simulink model "model"  (R2024a)
settings: Solver=ode4  StartTime=0.0  StopTime=6000  FixedStep=0.1  MaxStep=1  RelTol=1e-6  AbsTol=1e-9
undefined symbols (not defined in the file or in its folder): constants, P0, q0, rECI0, rSCI0, sensors, vECI0, vSCI0, w0
libraries: vrlib x2, aerolibatmos2 x1
settings Model: Creator=harryzhao  LastModifiedBy=harryzhao

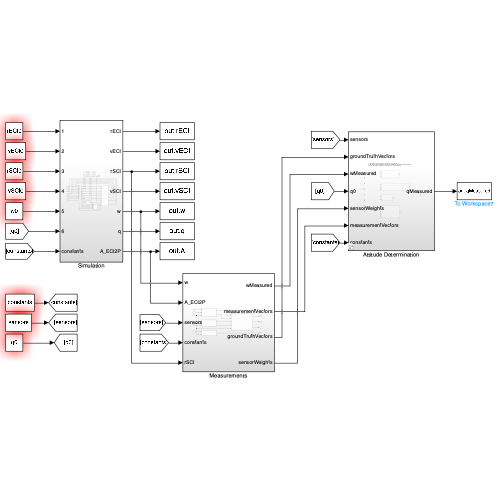
[thumbnail: Simulink's stored preview of the top-level diagram]
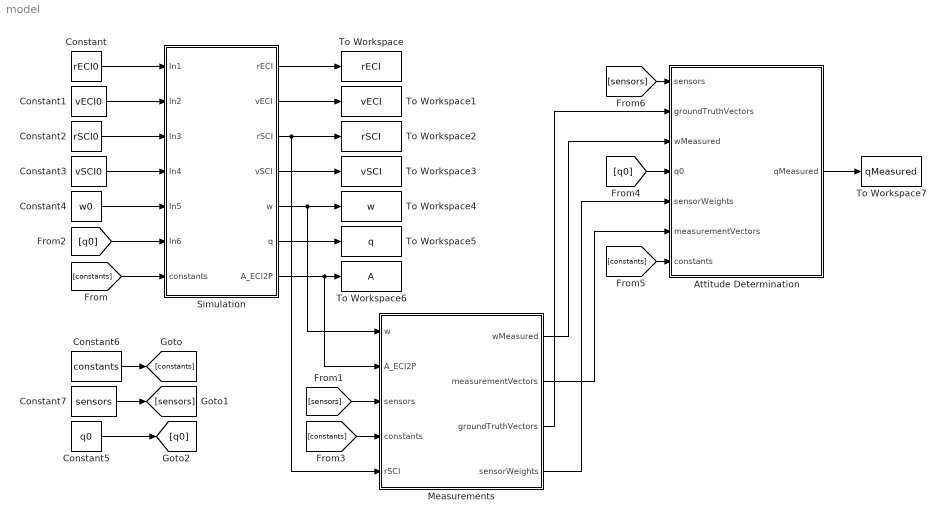
== system model ==
  Attitude Determination : Subsystem  Variant=on
  Constant : Constant  Value=rECI0
  Constant1 : Constant  Value=vECI0
  Constant2 : Constant  Value=rSCI0
  Constant3 : Constant  Value=vSCI0
  Constant4 : Constant  Value=w0
  Constant5 : Constant  Value=q0
  Constant6 : Constant  Value=constants  OutDataTypeStr=Bus: constants_bus
  Constant7 : Constant  Value=sensors  OutDataTypeStr=Bus: sensors_bus
  Measurements : Subsystem
  Simulation : Subsystem
  To Workspace : ToWorkspace  VariableName=rECI  SaveFormat=Timeseries  SampleTime=-1
  To Workspace1 : ToWorkspace  VariableName=vECI  SaveFormat=Timeseries  SampleTime=-1
  To Workspace2 : ToWorkspace  VariableName=rSCI  SaveFormat=Timeseries  SampleTime=-1
  To Workspace3 : ToWorkspace  VariableName=vSCI  SaveFormat=Timeseries  SampleTime=-1
  To Workspace4 : ToWorkspace  VariableName=w  SaveFormat=Timeseries  SampleTime=-1
  To Workspace5 : ToWorkspace  VariableName=q  SaveFormat=Timeseries  SampleTime=-1
  To Workspace6 : ToWorkspace  VariableName=A  SaveFormat=Timeseries  SampleTime=-1
  To Workspace7 : ToWorkspace  VariableName=qMeasured  SaveFormat=Timeseries  SampleTime=-1
  wires:
  Constant2/1 -> Simulation/3(In3)
  Measurements/4(sensorWeights) -> Attitude Determination/5(sensorWeights)
  Constant4/1 -> Simulation/5(In5)
  Measurements/2(measurementVectors) -> Attitude Determination/6(measurementVectors)
  Constant3/1 -> Simulation/4(In4)
  Simulation/1(rECI) -> To Workspace/1
  Simulation/2(vECI) -> To Workspace1/1
  Simulation/3(rSCI) -> Measurements/5(rSCI), To Workspace2/1
  Simulation/4(vSCI) -> To Workspace3/1
  Simulation/5(w) -> Measurements/1(w), To Workspace4/1
  Simulation/6(q) -> To Workspace5/1
  Simulation/7(A_ECI2P) -> Measurements/2(A_ECI2P), To Workspace6/1
  Measurements/1(wMeasured) -> Attitude Determination/3(wMeasured)
  Measurements/3(groundTruthVectors) -> Attitude Determination/2(groundTruthVectors)
  Attitude Determination/1(qMeasured) -> To Workspace7/1
  Constant/1 -> Simulation/1(In1)
  Constant1/1 -> Simulation/2(In2)
  [q0] -> Simulation/6(In6)
  [constants] -> Simulation/7(constants)
  Constant6/1 -> [constants]
  Constant7/1 -> [sensors]
  Constant5/1 -> [q0]
  [sensors] -> Measurements/3(sensors)
  [constants] -> Measurements/4(constants)
  [q0] -> Attitude Determination/4(q0)
  [constants] -> Attitude Determination/7(constants)
  [sensors] -> Attitude Determination/1(sensors)

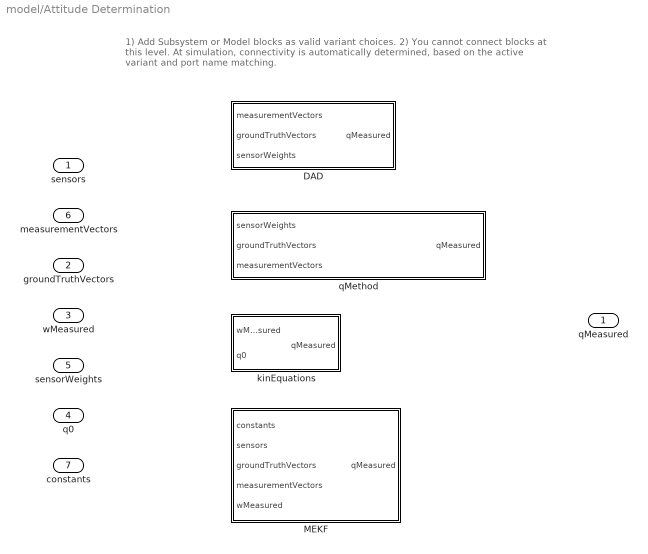
== system model/Attitude Determination ==
  note: 1) Add Subsystem or Model blocks as valid variant choices.
      | 2) You cannot connect blocks at this level. At simulation, connectivity is automatically
      | determined, based on the active variant and port name matching.
  sensors : Inport
  groundTruthVectors : Inport  Port=2
  wMeasured : Inport  Port=3
  q0 : Inport  Port=4
  sensorWeights : Inport  Port=5
  measurementVectors : Inport  Port=6
  constants : Inport  Port=7
  DAD : Subsystem  VariantControl="measType==\"dad\""
  MEKF : Subsystem  VariantControl="measType==\"MEKF\""
  kinEquations : Subsystem  VariantControl="measType==\"kin\""
  qMethod : Subsystem  VariantControl="measType==\"q\""
  qMeasured : Outport

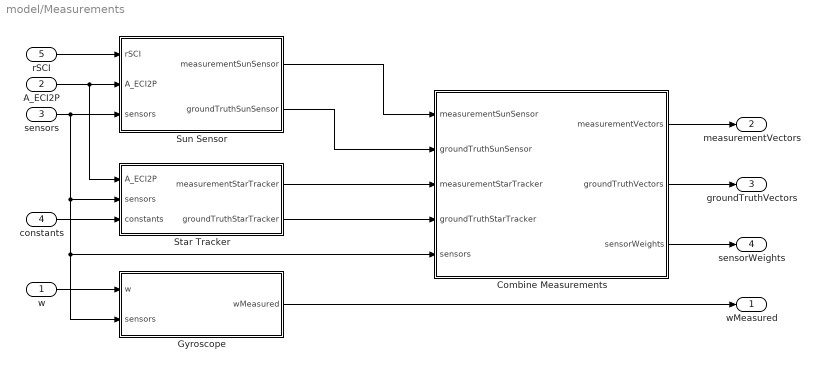
== system model/Measurements ==
  w : Inport
  A_ECI2P : Inport  Port=2
  sensors : Inport  Port=3
  constants : Inport  Port=4
  rSCI : Inport  Port=5
  Combine Measurements : MATLAB Function  TreatAsAtomicUnit=on
  Gyroscope : MATLAB Function  TreatAsAtomicUnit=on
  Star Tracker : MATLAB Function  TreatAsAtomicUnit=on
  Sun Sensor : MATLAB Function  TreatAsAtomicUnit=on
  wMeasured : Outport
  measurementVectors : Outport  Port=2
  groundTruthVectors : Outport  Port=3
  sensorWeights : Outport  Port=4
  wires:
  rSCI/1 -> Sun Sensor/1(rSCI)
  A_ECI2P/1 -> Star Tracker/1(A_ECI2P), Sun Sensor/2(A_ECI2P)
  sensors/1 -> Gyroscope/2(sensors), Combine Measurements/5(sensors), Star Tracker/2(sensors), Sun Sensor/3(sensors)
  constants/1 -> Star Tracker/3(constants)
  w/1 -> Gyroscope/1(w)
  Gyroscope/1(wMeasured) -> wMeasured/1
  Sun Sensor/2(groundTruthSunSensor) -> Combine Measurements/2(groundTruthSunSensor)
  Sun Sensor/1(measurementSunSensor) -> Combine Measurements/1(measurementSunSensor)
  Star Tracker/1(measurementStarTracker) -> Combine Measurements/3(measurementStarTracker)
  Star Tracker/2(groundTruthStarTracker) -> Combine Measurements/4(groundTruthStarTracker)
  Combine Measurements/1(measurementVectors) -> measurementVectors/1
  Combine Measurements/2(groundTruthVectors) -> groundTruthVectors/1
  Combine Measurements/3(sensorWeights) -> sensorWeights/1

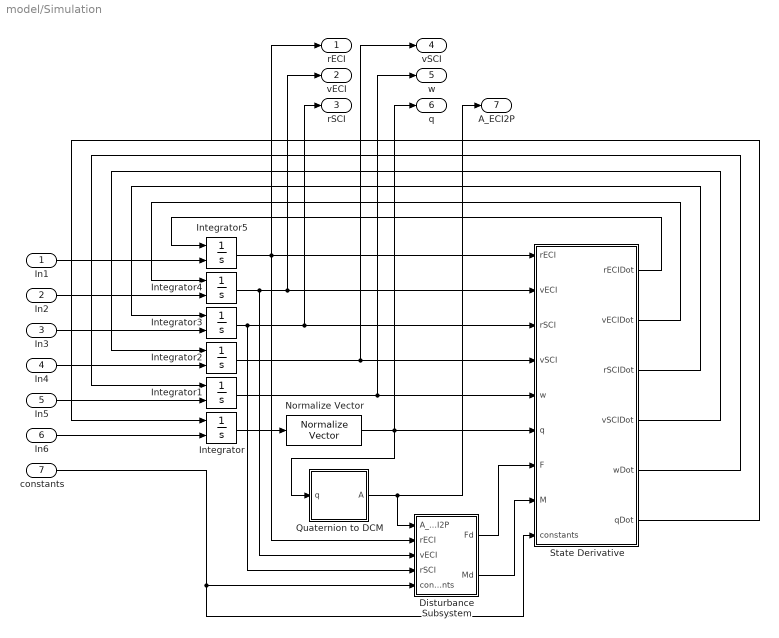
== system model/Simulation ==
  In1 : Inport
  In2 : Inport  Port=2
  In3 : Inport  Port=3
  In4 : Inport  Port=4
  In5 : Inport  Port=5
  In6 : Inport  Port=6
  constants : Inport  Port=7
  Disturbance Subsystem : Subsystem
  Integrator{,1..5} (6 alike) : Integrator  InitialConditionSource=external
  Normalize Vector : vrlib/Utilities/Normalize Vector  maxzero=0
  Quaternion to DCM : MATLAB Function  TreatAsAtomicUnit=on
  State Derivative : MATLAB Function  TreatAsAtomicUnit=on
  rECI : Outport
  vECI : Outport  Port=2
  rSCI : Outport  Port=3
  vSCI : Outport  Port=4
  w : Outport  Port=5
  q : Outport  Port=6
  A_ECI2P : Outport  Port=7
  wires:
  Disturbance Subsystem/1(Fd) -> State Derivative/7(F)
  Integrator3/1 -> rSCI/1, State Derivative/3(rSCI), Disturbance Subsystem/4(rSCI)
  Integrator2/1 -> vSCI/1, State Derivative/4(vSCI)
  Integrator/1 -> Normalize Vector/1
  In2/1 -> Integrator4/2
  Integrator5/1 -> rECI/1, State Derivative/1(rECI), Disturbance Subsystem/2(rECI)
  Normalize Vector/1 -> Quaternion to DCM/1(q), q/1, State Derivative/6(q)
  constants/1 -> Disturbance Subsystem/5(constants), State Derivative/9(constants)
  Integrator4/1 -> vECI/1, State Derivative/2(vECI), Disturbance Subsystem/3(vECI)
  In3/1 -> Integrator3/2
  State Derivative/3(rSCIDot) -> Integrator3/1
  State Derivative/1(rECIDot) -> Integrator5/1
  Quaternion to DCM/1(A) -> A_ECI2P/1, Disturbance Subsystem/1(A_ECI2P)
  State Derivative/4(vSCIDot) -> Integrator2/1
  Disturbance Subsystem/2(Md) -> State Derivative/8(M)
  State Derivative/6(qDot) -> Integrator/1
  Integrator1/1 -> w/1, State Derivative/5(w)
  State Derivative/5(wDot) -> Integrator1/1
  In4/1 -> Integrator2/2
  State Derivative/2(vECIDot) -> Integrator4/1
  In6/1 -> Integrator/2
  In5/1 -> Integrator1/2
  In1/1 -> Integrator5/2

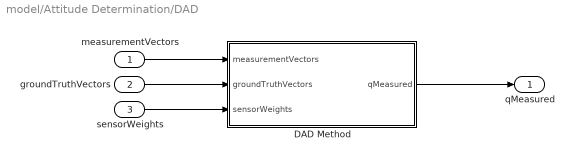
== system model/Attitude Determination/DAD ==
  measurementVectors : Inport
  groundTruthVectors : Inport  Port=2
  sensorWeights : Inport  Port=3
  DAD Method : Subsystem  Variant=on
  qMeasured : Outport
  wires:
  groundTruthVectors/1 -> DAD Method/2(groundTruthVectors)
  measurementVectors/1 -> DAD Method/1(measurementVectors)
  DAD Method/1(qMeasured) -> qMeasured/1
  sensorWeights/1 -> DAD Method/3(sensorWeights)

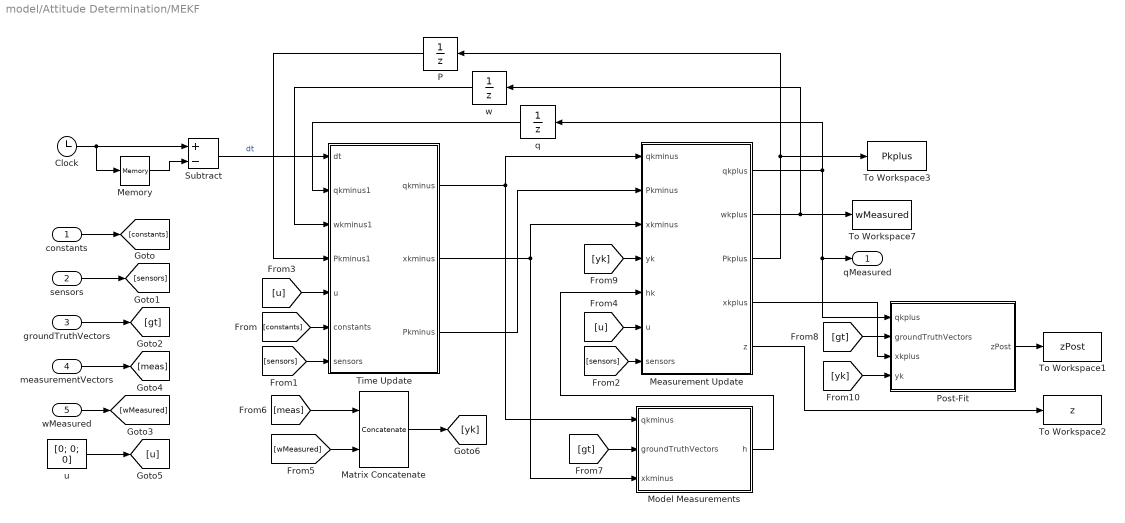
== system model/Attitude Determination/MEKF ==
  constants : Inport
  sensors : Inport  Port=2
  groundTruthVectors : Inport  Port=3
  measurementVectors : Inport  Port=4
  wMeasured : Inport  Port=5
  Clock : Clock
  Matrix Concatenate : Concatenate  Mode=Multidimensional array  ConcatenateDimension=2
  Measurement Update : MATLAB Function  TreatAsAtomicUnit=on
  Memory : Memory
  Model Measurements : Subsystem
  P : UnitDelay  InitialCondition=P0  SampleTime=-1  HasFrameUpgradeWarning=on
  Post-Fit : Subsystem
  Subtract : Sum  Inputs=+-
  Time Update : MATLAB Function  TreatAsAtomicUnit=on
  To Workspace1 : ToWorkspace  VariableName=zPost  SaveFormat=Timeseries  SampleTime=-1
  To Workspace2 : ToWorkspace  VariableName=z  SaveFormat=Timeseries  SampleTime=-1
  To Workspace3 : ToWorkspace  VariableName=Pkplus  SaveFormat=Timeseries  SampleTime=-1
  To Workspace7 : ToWorkspace  VariableName=wMeasured  SaveFormat=Timeseries  SampleTime=-1
  q : UnitDelay  InitialCondition=q0  SampleTime=-1  HasFrameUpgradeWarning=on
  u : Constant  Value=[0; 0; 0]
  w : UnitDelay  InitialCondition=w0'  SampleTime=-1  HasFrameUpgradeWarning=on
  qMeasured : Outport
  wires:
  Clock/1 -> Memory/1, Subtract/1
  Memory/1 -> Subtract/2
  Time Update/2(xkminus) -> Measurement Update/3(xkminus), Model Measurements/3(xkminus)
  Subtract/1 -> Time Update/1(dt)  "dt"
  Time Update/1(qkminus) -> Measurement Update/1(qkminus), Model Measurements/1(qkminus)
  Time Update/3(Pkminus) -> Measurement Update/2(Pkminus)
  Model Measurements/1(h) -> Measurement Update/5(hk)
  Measurement Update/1(qkplus) -> Post-Fit/1(qkplus), qMeasured/1, q/1
  Measurement Update/2(wkplus) -> To Workspace7/1, w/1
  Measurement Update/3(Pkplus) -> P/1, To Workspace3/1
  P/1 -> Time Update/4(Pkminus1)
  w/1 -> Time Update/3(wkminus1)
  q/1 -> Time Update/2(qkminus1)
  Measurement Update/4(xkplus) -> Post-Fit/3(xkplus)
  constants/1 -> [constants]
  sensors/1 -> [sensors]
  [constants] -> Time Update/6(constants)
  [sensors] -> Time Update/7(sensors)
  [sensors] -> Measurement Update/7(sensors)
  u/1 -> [u]
  [u] -> Time Update/5(u)
  [u] -> Measurement Update/6(u)
  wMeasured/1 -> [wMeasured]
  [wMeasured] -> Matrix Concatenate/2
  measurementVectors/1 -> [meas]
  [meas] -> Matrix Concatenate/1
  groundTruthVectors/1 -> [gt]
  [gt] -> Model Measurements/2(groundTruthVectors)
  [gt] -> Post-Fit/2(groundTruthVectors)
  Measurement Update/5(z) -> To Workspace2/1
  Matrix Concatenate/1 -> [yk]
  [yk] -> Measurement Update/4(yk)
  [yk] -> Post-Fit/4(yk)
  Post-Fit/1(zPost) -> To Workspace1/1

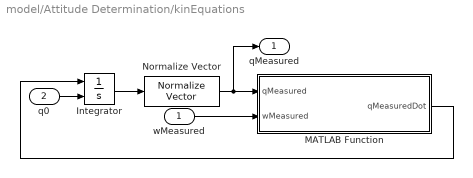
== system model/Attitude Determination/kinEquations ==
  wMeasured : Inport
  q0 : Inport  Port=2
  Integrator : Integrator  InitialConditionSource=external
  MATLAB Function : MATLAB Function  TreatAsAtomicUnit=on
  Normalize Vector : vrlib/Utilities/Normalize Vector  maxzero=0
  qMeasured : Outport
  wires:
  wMeasured/1 -> MATLAB Function/2(wMeasured)
  MATLAB Function/1(qMeasuredDot) -> Integrator/1
  q0/1 -> Integrator/2
  Normalize Vector/1 -> qMeasured/1, MATLAB Function/1(qMeasured)
  Integrator/1 -> Normalize Vector/1

== system model/Attitude Determination/qMethod ==
  sensorWeights : Inport
  groundTruthVectors : Inport  Port=2
  measurementVectors : Inport  Port=3
  MATLAB Function : MATLAB Function  TreatAsAtomicUnit=on
  qMeasured : Outport
  wires:
  MATLAB Function/1(qMeasured) -> qMeasured/1
  sensorWeights/1 -> MATLAB Function/3(sensorWeights)
  groundTruthVectors/1 -> MATLAB Function/2(groundTruthVectors)
  measurementVectors/1 -> MATLAB Function/1(measurementVectors)

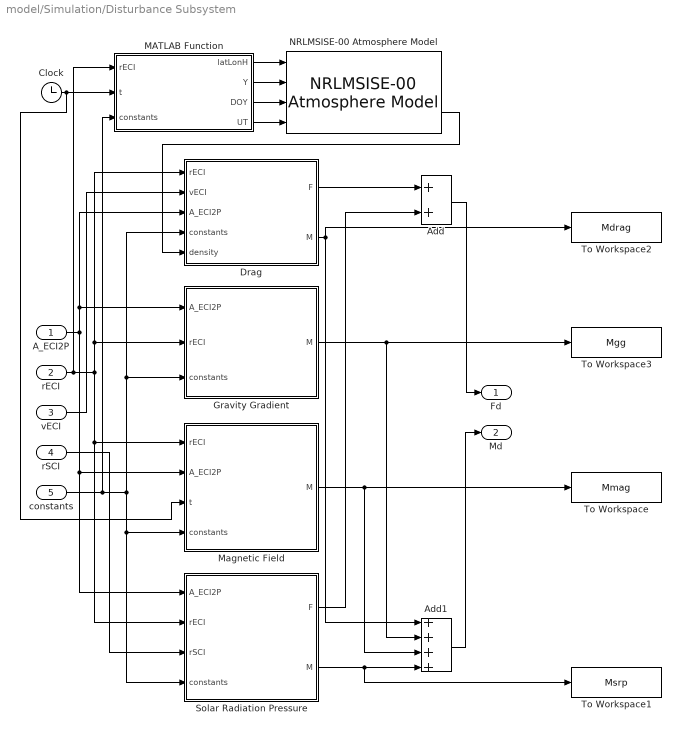
== system model/Simulation/Disturbance Subsystem ==
  A_ECI2P : Inport
  rECI : Inport  Port=2
  vECI : Inport  Port=3
  rSCI : Inport  Port=4
  constants : Inport  Port=5
  Add : Sum
  Add1 : Sum  Inputs=++++
  Clock : Clock
  Drag : MATLAB Function  TreatAsAtomicUnit=on
  Gravity Gradient : MATLAB Function  TreatAsAtomicUnit=on
  MATLAB Function : MATLAB Function  TreatAsAtomicUnit=on
  Magnetic Field : MATLAB Function  TreatAsAtomicUnit=on
  NRLMSISE-00 Atmosphere Model : aerolibatmos2/NRLMSISE-00 Atmosphere Model  units=Metric (MKS)  lst_input=off  flux_ap_input=off  flags_input=Internal  flags=ones(1,23)  oxygen_in=off  action=Warning
  Solar Radiation Pressure : MATLAB Function  TreatAsAtomicUnit=on
  To Workspace : ToWorkspace  VariableName=Mmag  SaveFormat=Timeseries  SampleTime=-1
  To Workspace1 : ToWorkspace  VariableName=Msrp  SaveFormat=Timeseries  SampleTime=-1
  To Workspace2 : ToWorkspace  VariableName=Mdrag  SaveFormat=Timeseries  SampleTime=-1
  To Workspace3 : ToWorkspace  VariableName=Mgg  SaveFormat=Timeseries  SampleTime=-1
  Fd : Outport
  Md : Outport  Port=2
  wires:
  Gravity Gradient/1(M) -> To Workspace3/1, Add1/2
  Drag/2(M) -> To Workspace2/1, Add1/1
  Solar Radiation Pressure/1(F) -> Add/2
  Drag/1(F) -> Add/1
  Add/1 -> Fd/1
  Add1/1 -> Md/1
  A_ECI2P/1 -> Magnetic Field/2(A_ECI2P), Solar Radiation Pressure/1(A_ECI2P), Drag/3(A_ECI2P), Gravity Gradient/1(A_ECI2P)
  rECI/1 -> MATLAB Function/1(rECI), Solar Radiation Pressure/2(rECI), Magnetic Field/1(rECI), Gravity Gradient/2(rECI), Drag/1(rECI)
  vECI/1 -> Drag/2(vECI)
  rSCI/1 -> Solar Radiation Pressure/3(rSCI)
  Solar Radiation Pressure/2(M) -> To Workspace1/1, Add1/4
  Magnetic Field/1(M) -> To Workspace/1, Add1/3
  constants/1 -> MATLAB Function/3(constants), Magnetic Field/4(constants), Solar Radiation Pressure/4(constants), Gravity Gradient/3(constants), Drag/4(constants)
  MATLAB Function/2(Y) -> NRLMSISE-00 Atmosphere Model/2
  MATLAB Function/3(DOY) -> NRLMSISE-00 Atmosphere Model/3
  MATLAB Function/4(UT) -> NRLMSISE-00 Atmosphere Model/4
  MATLAB Function/1(latLonH) -> NRLMSISE-00 Atmosphere Model/1
  NRLMSISE-00 Atmosphere Model/2 -> Drag/5(density)
  Clock/1 -> MATLAB Function/2(t), Magnetic Field/3(t)

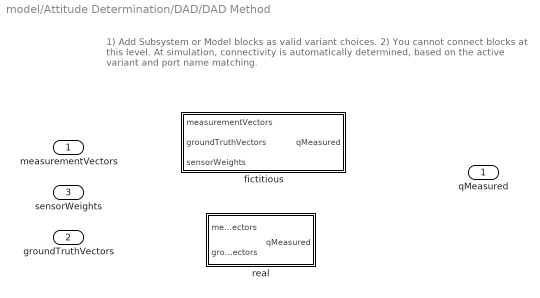
== system model/Attitude Determination/DAD/DAD Method ==
  note: 1) Add Subsystem or Model blocks as valid variant choices.
      | 2) You cannot connect blocks at this level. At simulation, connectivity is automatically
      | determined, based on the active variant and port name matching.
  measurementVectors : Inport
  groundTruthVectors : Inport  Port=2
  sensorWeights : Inport  Port=3
  fictitious : Subsystem  VariantControl=useFict == true
  real : Subsystem  VariantControl=useFict == false
  qMeasured : Outport

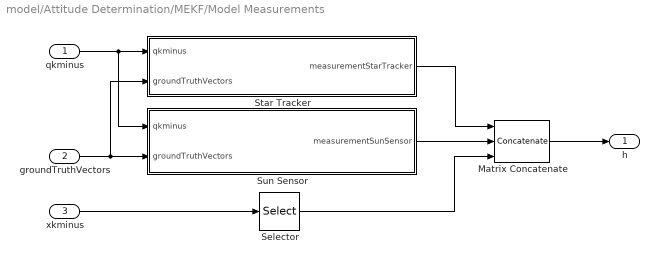
== system model/Attitude Determination/MEKF/Model Measurements ==
  qkminus : Inport
  groundTruthVectors : Inport  Port=2
  xkminus : Inport  Port=3
  Matrix Concatenate : Concatenate  NumInputs=3  Mode=Multidimensional array  ConcatenateDimension=2
  Selector : Selector  NumberOfDimensions=2  InputPortWidth=3  IndexOptions=Index vector (dialog),Index vector (dialog)  Indices=[4:6],1  OutputSizes=1,1
  Star Tracker : MATLAB Function  TreatAsAtomicUnit=on
  Sun Sensor : MATLAB Function  TreatAsAtomicUnit=on
  h : Outport
  wires:
  groundTruthVectors/1 -> Star Tracker/2(groundTruthVectors), Sun Sensor/2(groundTruthVectors)
  qkminus/1 -> Sun Sensor/1(qkminus), Star Tracker/1(qkminus)
  Star Tracker/1(measurementStarTracker) -> Matrix Concatenate/1
  Sun Sensor/1(measurementSunSensor) -> Matrix Concatenate/2
  Matrix Concatenate/1 -> h/1
  xkminus/1 -> Selector/1
  Selector/1 -> Matrix Concatenate/3

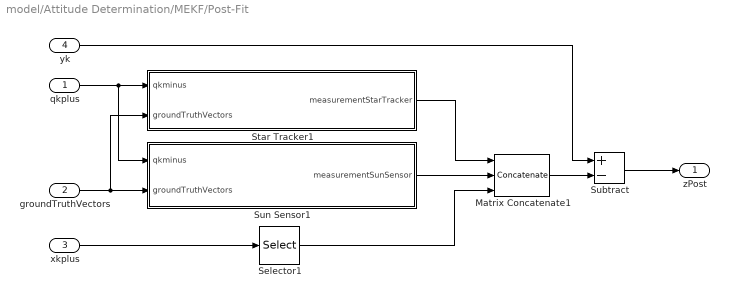
== system model/Attitude Determination/MEKF/Post-Fit ==
  qkplus : Inport
  groundTruthVectors : Inport  Port=2
  xkplus : Inport  Port=3
  yk : Inport  Port=4
  Matrix Concatenate1 : Concatenate  NumInputs=3  Mode=Multidimensional array  ConcatenateDimension=2
  Selector1 : Selector  NumberOfDimensions=2  InputPortWidth=3  IndexOptions=Index vector (dialog),Index vector (dialog)  Indices=[4:6],1  OutputSizes=1,1
  Star Tracker1 : MATLAB Function  TreatAsAtomicUnit=on
  Subtract : Sum  Inputs=+-
  Sun Sensor1 : MATLAB Function  TreatAsAtomicUnit=on
  zPost : Outport
  wires:
  Subtract/1 -> zPost/1
  qkplus/1 -> Sun Sensor1/1(qkminus), Star Tracker1/1(qkminus)
  Selector1/1 -> Matrix Concatenate1/3
  xkplus/1 -> Selector1/1
  groundTruthVectors/1 -> Star Tracker1/2(groundTruthVectors), Sun Sensor1/2(groundTruthVectors)
  Star Tracker1/1(measurementStarTracker) -> Matrix Concatenate1/1
  Sun Sensor1/1(measurementSunSensor) -> Matrix Concatenate1/2
  Matrix Concatenate1/1 -> Subtract/2
  yk/1 -> Subtract/1

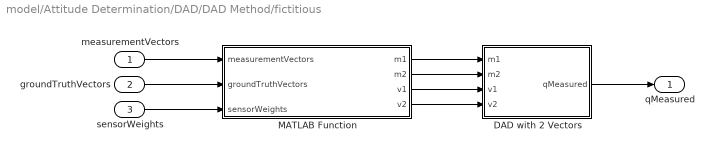
== system model/Attitude Determination/DAD/DAD Method/fictitious ==
  measurementVectors : Inport
  groundTruthVectors : Inport  Port=2
  sensorWeights : Inport  Port=3
  DAD with 2 Vectors : MATLAB Function  TreatAsAtomicUnit=on
  MATLAB Function : MATLAB Function  TreatAsAtomicUnit=on
  qMeasured : Outport
  wires:
  measurementVectors/1 -> MATLAB Function/1(measurementVectors)
  groundTruthVectors/1 -> MATLAB Function/2(groundTruthVectors)
  MATLAB Function/1(m1) -> DAD with 2 Vectors/1(m1)
  MATLAB Function/2(m2) -> DAD with 2 Vectors/2(m2)
  MATLAB Function/3(v1) -> DAD with 2 Vectors/3(v1)
  MATLAB Function/4(v2) -> DAD with 2 Vectors/4(v2)
  DAD with 2 Vectors/1(qMeasured) -> qMeasured/1
  sensorWeights/1 -> MATLAB Function/3(sensorWeights)

== system model/Attitude Determination/DAD/DAD Method/real ==
  measurementVectors : Inport
  groundTruthVectors : Inport  Port=2
  MATLAB Function : MATLAB Function  TreatAsAtomicUnit=on
  qMeasured : Outport
  wires:
  measurementVectors/1 -> MATLAB Function/1(measurementVectors)
  groundTruthVectors/1 -> MATLAB Function/2(groundTruthVectors)
  MATLAB Function/1(qMeasured) -> qMeasured/1

== matlab function model/Attitude Determination/DAD/DAD Method/fictitious/DAD with 2 Vectors ==
  data: m1 input; qMeasured output; m2 input; v1 input; v2 input
function qMeasured = DAD2Vec(m1, m2, v1, v2)
% Implement the Deterministic Atittude Determination algorithm
% Inputs:
% - m1, m2: measured vectors
% - v1, v2: ground truth vector
% Outputs:
% - A: DCM between principal axes and ECI

pm = m1;
cross_qm = cross(m1, m2);
qm = cross_qm/norm(cross_qm);
rm = cross(pm, qm);

pv = v1;
cross_qv = cross(v1, v2);
qv = cross_qv/norm(cross_qv);
rv = cross(pv,qv);

M = [pm qm rm];
V = [pv qv rv];
A = M / V;
qMeasured = A2q(A);
end

== matlab function model/Attitude Determination/qMethod/MATLAB Function ==
  data: measurementVectors input; groundTruthVectors input; sensorWeights input; qMeasured output size=[4, 1]
function qMeasured = qMethod(measurementVectors, groundTruthVectors, sensorWeights)
    % Implement the Deterministic q method
    % Inputs:
    % - m: measured vectors
    % - v: ground truth vector
    % - w: weights of sensor measurements
    % Outputs:
    % - A: DCM between principal axes and ECI

    % Get data from sensors
    m = measurementVectors;
    v = groundTruthVectors;
    w = sensorWeights;
    % m = ones(3); v = ones(3); w = ones(3);


    U = sqrt(w) .* v;
    W = sqrt(w) .* m;

    B = W * U';
    S = B + B';
    Z = [B(2,3)-B(3,2), B(3,1)-B(1,3), B(1,2)-B(2,1)]';
    sigma = trace(B);

    K = [S - eye(size(S))*sigma, Z;
            Z', sigma];

    [V, lamda] = eig(K);

    [~, nMax] = max(diag(lamda));

    qMeasured = V(:, nMax);
    qMeasured = A2q(q2A(qMeasured));
end

== matlab function model/Attitude Determination/kinEquations/MATLAB Function ==
  data: qMeasured input; qMeasuredDot output; wMeasured input
function qMeasuredDot = kinQuats(qMeasured, wMeasured)
    
    w = wMeasured;

    sigma = [0, w(3), -w(2), w(1); ...
        -w(3), 0, w(1), w(2); ...
        w(2), -w(1), 0, w(3); ...
        -w(1), -w(2), -w(3), 0];
    qMeasuredDot = 0.5 * sigma * qMeasured;
end

== matlab function model/Attitude Determination/DAD/DAD Method/fictitious/MATLAB Function ==
  data: measurementVectors input; m1 output; groundTruthVectors input; m2 output; v1 output; v2 output; sensorWeights input
function [m1, m2, v1, v2] = getMeasurementsFict(measurementVectors, groundTruthVectors, sensorWeights)
    [~, indBest2Sensors] = maxk(sensorWeights, 2);
    mVec = measurementVectors(:,indBest2Sensors);
    vVec = groundTruthVectors(:,indBest2Sensors);

    m1 = (mVec(:,1) + mVec(:,2))/2;
    m2 = (mVec(:,1) - mVec(:,2))/2;
    v1 = (vVec(:,1) + vVec(:,2))/2;
    v2 = ((vVec(:,1) - vVec(:,2))/2);

    m1 = m1 / norm(m1);
    m2 = m2 / norm(m2);
    v1 = v1 / norm(v1);
    v2 = v2 / norm(v2);
end

== matlab function model/Attitude Determination/DAD/DAD Method/real/MATLAB Function ==
  data: measurementVectors input; qMeasured output; groundTruthVectors input
function qMeasured = DAD(measurementVectors, groundTruthVectors)
    % Implement the Deterministic Atittude Determination algorithm
    % Inputs:
    % - m: measured vectors ([m1 m2 . . . ])
    % - v: ground truth vector ([v1 v2 . . . ])
    % Outputs:
    % - A: DCM between principal axes and ECI

    A = measurementVectors * pinv(groundTruthVectors);
    qMeasured = A2q(A);
end

== matlab function model/Measurements/Sun Sensor ==
  settings: updateMethod=DISCRETE
  data: rSCI input; A_ECI2P input; sensors input; measurementSunSensor output; groundTruthSunSensor output
function [measurementSunSensor,groundTruthSunSensor] = sunSensor(rSCI, A_ECI2P, sensors)
    % Get sensor measurement without noise
    rSunSensors = A_ECI2P * rSCI;
    rSunSensors = normVec(rSunSensors);
    
    % Add noise
    % measurementSunSensor = addVectorNoise(rSunSensors, sensors.sunError);
    measurementSunSensor = addNoise(rSunSensors, sensors.sunError);
    measurementSunSensor = normVec(measurementSunSensor);

    % Get groud truth
    groundTruthSunSensor = normVec(rSCI);

end

== matlab function model/Measurements/Star Tracker ==
  settings: updateMethod=DISCRETE
  data: A_ECI2P input; sensors input; constants input; measurementStarTracker output; groundTruthStarTracker output
function [measurementStarTracker, groundTruthStarTracker] = starTracker(A_ECI2P, sensors, constants)
    % Get sensor measurement without noise (body axes)
    % numStars = sensors.numStars;
    numStars = 10;
    rStarBody = zeros([3, numStars*2]);
    for i = 1:numStars
        theta = deg2rad(randi([0 359], 1));
        phi = 2*sensors.trackerFOV *rand(1) - sensors.trackerFOV;
        rStarBody(:,i) = [cos(theta)*sin(phi); cos(phi); sin(theta)*sin(phi)];
        rStarBody(:,i+numStars) = [cos(theta)*sin(phi); -cos(phi); sin(theta)*sin(phi)];
    end

    % Convert to principal axes
    rStarP = constants.A_Body2P * rStarBody;

    measurementStarTracker = addNoise(rStarP, sensors.trackerError);
    measurementStarTracker = normVec(measurementStarTracker);

    % Get ground truth data
    groundTruthStarTracker = A_ECI2P' * rStarP;
end

== matlab function model/Measurements/Gyroscope ==
  settings: updateMethod=DISCRETE
  data: w input; sensors input; wMeasured output
function wMeasured = gyro(w, sensors)
    % Add noise to gyro measurements
    wMeasured = addNoise(w, sensors.gyroError, sensors.gyroBias);
end

== matlab function model/Measurements/Combine Measurements ==
  data: measurementSunSensor input; groundTruthSunSensor input; measurementStarTracker input; groundTruthStarTracker input; sensors input; measurementVectors output; groundTruthVectors output; sensorWeights output
function [measurementVectors, groundTruthVectors, sensorWeights] = concatenateMeasurements(measurementSunSensor, groundTruthSunSensor, measurementStarTracker, groundTruthStarTracker, sensors)
    % Initialize
    vectorSize = size(measurementStarTracker, 2) + size(measurementSunSensor, 2);

    % Concatenate such that we have [starTracker, sunSensor]
    measurementVectors = [measurementStarTracker, measurementSunSensor];
    groundTruthVectors = [groundTruthStarTracker, groundTruthSunSensor];
    
    % Get sensor weighting
    sensorWeights = [ones([1, vectorSize-1])*sensors.weights(1), sensors.weights(2)];
end

== matlab function model/Attitude Determination/MEKF/Post-Fit/Star Tracker1 ==
  settings: updateMethod=DISCRETE
  data: qkminus input; groundTruthVectors input; measurementStarTracker output
function measurementStarTracker = starTracker(qkminus,groundTruthVectors)
    % Extract information
    A_ECI2P = q2A(qkminus);
    rStarECI = groundTruthVectors(:,1:end-1);
    rStarP = A_ECI2P * rStarECI;

    measurementStarTracker = normVec(rStarP);
end

== matlab function model/Attitude Determination/MEKF/Post-Fit/Sun Sensor1 ==
  settings: updateMethod=DISCRETE
  data: qkminus input; groundTruthVectors input; measurementSunSensor output
function measurementSunSensor = sunSensor(qkminus,groundTruthVectors)
    % Get modeled parameters
    rSCI = groundTruthVectors(:,end);
    A_ECI2P = q2A(qkminus);

    % Get sensor measurement without noise
    rSunSensors = A_ECI2P * rSCI;
    measurementSunSensor = normVec(rSunSensors);
end

== matlab function model/Attitude Determination/MEKF/Measurement Update ==
  data: qkminus input; Pkminus input; xkminus input; yk input; hk input; u input; sensors input; qkplus output; wkplus output; Pkplus output; xkplus output; z output
function [qkplus,wkplus,Pkplus,xkplus,z] = measurementUpdate(qkminus, Pkminus, xkminus, yk, hk, u, sensors)
    % Get R
    numVectMeasurements = size(hk,2)-1;
    R = diag([repelem(sensors.trackerError, 3*(numVectMeasurements-1)), repelem(sensors.sunError, 3), repelem(sensors.gyroError, 3)]).^2;

    % Compute residual
    z = yk - hk;

    % Adjust yk and hk vectors
    yk = yk(:);
    hk = hk(:);
    
    % Get Hk
    Hk = zeros([3*(numVectMeasurements+1), 6]);
    for n = 1:3:(3*numVectMeasurements)
        Hk_vect = crossMatrix(hk(n:n+2));
        Hk(n:n+2,:) = [Hk_vect, zeros(3)];
    end
    Hk(end-2:end,:) = [zeros(3), eye(3)];
    Kk = (Pkminus * Hk') / (Hk * Pkminus * Hk' + R);
    xkplus = xkminus + Kk * (yk - hk);
    Pkplus = Pkminus - Kk * Hk * Pkminus;
    wkplus = xkplus(4:6);
    ax = xkplus(1); ay = xkplus(2); az = xkplus(3);

    % Attitude update
    qkplus = [1, az/2, -ay/2, ax/2; ...
        -az/2, 1, ax/2, ay/2; ...
        ay/2, -ax/2, 1, az/2; ...
        -ax/2, -ay/2, -az/2, 1] * qkminus;
end

== matlab function model/Simulation/Quaternion to DCM ==
  data: q input size=[4 1]; A output
function A = q2A(q)
    q1 = q(1); q2 = q(2); q3 = q(3); q0 = q(4);
    A = [(q0^2 + q1^2 - q2^2 - q3^2) (2 * q1 * q2 + 2 * q0 * q3) (2 * q1 * q3 - 2 * q0 * q2); ...
        (2 * q1 * q2 - 2 * q0 * q3) (q0^2 - q1^2 + q2^2 - q3^2) (2 * q2 * q3 + 2 * q0 * q1); ...
        (2 * q1 * q3 + 2 * q0 * q2) (2 * q2 * q3 - 2 * q0 * q1) (q0^2 - q1^2 - q2^2 + q3^2)];
end

== matlab function model/Attitude Determination/MEKF/Model Measurements/Star Tracker ==
  settings: updateMethod=DISCRETE
  data: qkminus input; groundTruthVectors input; measurementStarTracker output
function measurementStarTracker = starTracker(qkminus,groundTruthVectors)
    % Extract information
    A_ECI2P = q2A(qkminus);
    rStarECI = groundTruthVectors(:,1:end-1);
    rStarP = A_ECI2P * rStarECI;

    measurementStarTracker = normVec(rStarP);
end

== matlab function model/Attitude Determination/MEKF/Model Measurements/Sun Sensor ==
  settings: updateMethod=DISCRETE
  data: qkminus input; groundTruthVectors input; measurementSunSensor output
function measurementSunSensor = sunSensor(qkminus,groundTruthVectors)
    % Get modeled parameters
    rSCI = groundTruthVectors(:,end);
    A_ECI2P = q2A(qkminus);

    % Get sensor measurement without noise
    rSunSensors = A_ECI2P * rSCI;
    measurementSunSensor = normVec(rSunSensors);
end

== matlab function model/Attitude Determination/MEKF/Time Update ==
  data: dt input; qkminus output size=[4, 1]; qkminus1 input; wkminus1 input; Pkminus1 input; u input; constants input; sensors input; xkminus output size=[6, 1]; Pkminus output size=[6, 6]
function [qkminus, xkminus, Pkminus] = timeUpdate(dt, qkminus1, wkminus1, Pkminus1, u, constants, sensors)
    % MEKF, only time update implemented

    % Get values
    Ix = constants.Ix; Iy = constants.Iy; Iz = constants.Iz;
    Q = sensors.Q;
    xkminus1 = [zeros([3 1]); wkminus1];

    w = norm(wkminus1);
    wcross = [0, -wkminus1(3), wkminus1(2); ...
        wkminus1(3), 0, -wkminus1(1); ...
        -wkminus1(2), wkminus1(1), 0];
    cw = cos(w * dt / 2);
    sw = sin(w * dt / 2);

    A = eye(3) + sw * wcross / w + (1 - cw) * wcross^2 / w^2;
    phi = eye(3) + 0.5 * dt * ...
        [0, (Iy - Iz) / Ix * wkminus1(3), (Iy - Iz) / Ix * wkminus1(2); ...
        (Iz - Ix) / Iy * wkminus1(3), 0, (Iz - Ix) / Iy * wkminus1(1); ...
        (Ix - Iy) / Iz * wkminus1(2), (Ix - Iy) / Iz * wkminus1(1), 0];
    B = dt * [1 / Ix, 0, 0; ...
        0, 1 / Iy, 0; ...
        0, 0, 1 / Iz];
    STM = [A, zeros(3); zeros(3), phi];
    O = eye(4) + 0.5 * dt * ...
        [0, wkminus1(3), -wkminus1(2), wkminus1(1); ...
        -wkminus1(3), 0, wkminus1(1), wkminus1(2); ...
        wkminus1(2), -wkminus1(1), 0, wkminus1(3); ...
        -wkminus1(1), -wkminus1(2), -wkminus1(3), 0];

    xkminus = STM * xkminus1 + [zeros([3 1]); B * u];
    wkminus = xkminus(4:6);
    qkminus = O * qkminus1;
    qkminus = normVec(qkminus);
    Pkminus = STM * Pkminus1 * STM' + Q;
end

== matlab function model/Simulation/State Derivative ==
  data: rECI input; rECIDot output; vECI input; rSCI input; vSCI input; w input; q input; F input; M input; constants input; vECIDot output; rSCIDot output; vSCIDot output; wDot output; qDot output
function [rECIDot,vECIDot,rSCIDot,vSCIDot,wDot,qDot] = ...
    timeDerivative(rECI,vECI,rSCI,vSCI,w,q,F,M,constants)

    % Satellite orbit around Earth
    rECIDot = vECI;
    vECIDot = (-3.986E5 / norm(rECI)^2) * rECI / norm(rECI); % km/s^2

    % Earth orbit around Sun
    rSCIDot = vSCI;
    vSCIDot = (-1.327E11 / norm(rSCI)^2) * ...
        rSCI / norm(rSCI); % km/s^2

    % Angular velocity
    wDot = zeros([3 1]);
    wDot(1) = (M(1) - ...
        (constants.Iz - constants.Iy) * w(2) * w(3)) / constants.Ix;
    wDot(2) = (M(2) - ...
        (constants.Ix - constants.Iz) * w(3) * w(1)) / constants.Iy;
    wDot(3) = (M(3) - ...
        (constants.Iy - constants.Ix) * w(1) * w(2)) / constants.Iz;

    % Quarternions
    sigma = [0, w(3), -w(2), w(1); ...
        -w(3), 0, w(1), w(2); ...
        w(2), -w(1), 0, w(3); ...
        -w(1), -w(2), -w(3), 0];
    qDot = 0.5 * sigma * q;
end

== matlab function model/Simulation/Disturbance Subsystem/Solar Radiation Pressure ==
  data: A_ECI2P input; F output; rECI input; rSCI input; constants input; M output
function [F,M] = SRP(A_ECI2P,rECI,rSCI,constants)
    % Earth axial tilt hard-coded
    Rx = [1 0 0; 0 cosd(23.5) -sind(23.5); 0 sind(23.5) cosd(23.5)];
    s = A_ECI2P * (-Rx * rSCI - rECI); % SCI -> ECI -> XYZ
    u = s / norm(s);
    N = constants.normal;
    Aeff = ((u' * N) > 0) .* constants.area;
    rC = constants.barycenter - constants.cm;
    theta = acos((u' * N) ./ (norm(u) * vecnorm(N)));
    SRP = -constants.P * cos(theta) .* Aeff .* ...
        ((1 - constants.Cs) * u + 2 * ...
        (constants.Cs * cos(theta) + constants.Cd / 3) .* N);
    F = sum(SRP,2);
    M = sum(cross(rC,SRP),2);
end

== matlab function model/Simulation/Disturbance Subsystem/Drag ==
  data: rECI input; F output; vECI input; A_ECI2P input; constants input; M output; density input
function [F,M] = drag(rECI,vECI,A_ECI2P,constants,density)
    % [~,density] = atmosnrlmsise00(1000 * (norm(rECI) - 6378.1),0,0,2000,1,0);
    rho = density(6);
    vP = A_ECI2P * (vECI + cross([0; 0; 7.2921159E-5],rECI));
    u = vP / norm(vP);
    N = constants.normal;
    Aeff = ((u' * N) > 0) .* constants.area;
    rC = constants.barycenter - constants.cm;
    D = -0.5 * constants.CD * rho * norm(vP)^2 * (u' * (N .* Aeff)) .* u;
    F = sum(D,2);
    M = sum(cross(rC,D),2);
end

== matlab function model/Simulation/Disturbance Subsystem/Gravity Gradient ==
  data: A_ECI2P input; rECI input; M output; constants input
function M = gravGrad(A_ECI2P,rECI,constants)
    radial = rECI / norm(rECI);
    c = A_ECI2P * radial;
    cx = c(1);
    cy = c(2);
    cz = c(3);
    M = zeros([3 1]);
    M(1) = 3 * constants.n^2 * (constants.Iz - constants.Iy) * cy * cz;
    M(2) = 3 * constants.n^2 * (constants.Ix - constants.Iz) * cz * cx;
    M(3) = 3 * constants.n^2 * (constants.Iy - constants.Ix) * cx * cy;
end

== matlab function model/Simulation/Disturbance Subsystem/Magnetic Field ==
  data: rECI input; A_ECI2P input; t input; constants input; M output
function M = mag(rECI,A_ECI2P,t,constants)
    % Calculated the expected torque due to Earth's magnetic field
    % Inputs:
    % - m: magnetic moment of satellite [N * m / T]
    % - R: position vector of satellite [km]
    % - t: time of simulation [s]
    % - RE: radius of Earth [km] (6378 km)
    % - UT1: start time of simulation

    GMST = time2GMST(t,UT12MJD(constants.UT1));
    [lat,lon,~] = ECEF2Geoc(ECI2ECEF(rECI,GMST),t);
    theta = pi/2 - lat;

    [B_R,B_theta,B_phi] = magFieldEarth(rECI,lon,theta,constants.RE);

    delta = lat;
    alpha = lon + GMST;

    B_x = (B_R * cos(delta) + B_theta * sin(delta)) * ...
        cos(alpha) - B_phi * sin(alpha);
    B_y = (B_R * cos(delta) + B_theta * sin(delta)) * ...
        sin(alpha) + B_phi * cos(alpha);
    B_z = (B_R * sin(delta) - B_theta * cos(delta));

    B_ECI = [B_x;B_y;B_z];
    B = A_ECI2P * B_ECI;

    M = cross(constants.m,B);
end

== matlab function model/Simulation/Disturbance Subsystem/MATLAB Function ==
  data: latLonH output; rECI input; t input; constants input; Y output; DOY output; UT output
function [latLonH,Y,DOY,UT] = atmHelper(rECI,t,constants)
    % Get time info
    UT1 = constants.UT1;
    Y = UT1(1);
    DOY = UT1(2);
    UT = UT1(3);

    % Get lat/long info
    GMST = time2GMST(t,UT12MJD(constants.UT1));
    [lat,lon,~] = ECEF2Geoc(ECI2ECEF(rECI,GMST),t);
    h = 1000*(norm(rECI) - constants.RE);
    latLonH = [rad2deg(lat), rad2deg(lon), h];
end
